simulink model "eight_point_dft"  (R2018a)
settings: Solver=VariableStepAuto  StartTime=0.0  StopTime=10.0  RelTol=1e-3
undefined symbols (not defined in the file): j
settings Model: Creator=eechris  LastModifiedBy=eechris

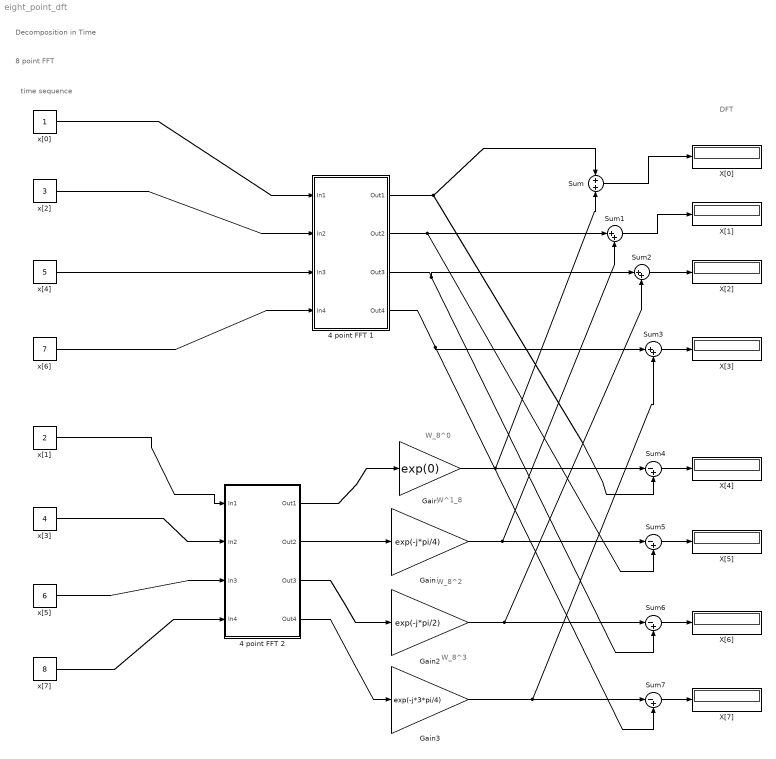
== system eight_point_dft ==
  note: Decomposition in Time
  note: W_8^3
  note: W_8^2
  note: W^1_8
  note: W_8^0
  note: time sequence
  note: DFT
  note: 8 point FFT
  4 point FFT 1 : Subsystem
  4 point FFT 2 : Subsystem
  Gain : Gain  Gain=exp(0)
  Gain1 : Gain  Gain=exp(-j*pi/4)
  Gain2 : Gain  Gain=exp(-j*pi/2)
  Gain3 : Gain  Gain=exp(-j*3*pi/4)
  Sum : Sum  Inputs=+|+
  Sum1 : Sum  Inputs=|++
  Sum2 : Sum  Inputs=|++
  Sum3 : Sum  Inputs=|++
  Sum{4..7} (4 alike) : Sum  Inputs=|-+
  X[0] : Display
  X[1] : Display
  X[2] : Display
  X[3] : Display
  X[4] : Display
  X[5] : Display
  X[6] : Display
  X[7] : Display
  x[0] : Constant
  x[1] : Constant  Value=2
  x[2] : Constant  Value=3
  x[3] : Constant  Value=4
  x[4] : Constant  Value=5
  x[5] : Constant  Value=6
  x[6] : Constant  Value=7
  x[7] : Constant  Value=8
  wires:
  x[0]/1 -> 4 point FFT 1/1(In1)
  x[7]/1 -> 4 point FFT 2/4(In4)
  Sum/1 -> X[0]/1
  4 point FFT 1/2(Out2) -> Sum5/2, Sum1/1
  Sum1/1 -> X[1]/1
  Sum3/1 -> X[3]/1
  Sum2/1 -> X[2]/1
  Sum4/1 -> X[4]/1
  Sum5/1 -> X[5]/1
  Sum6/1 -> X[6]/1
  Sum7/1 -> X[7]/1
  4 point FFT 2/1(Out1) -> Gain/1
  Gain/1 -> Sum/2, Sum4/1
  4 point FFT 2/2(Out2) -> Gain1/1
  Gain1/1 -> Sum1/2, Sum5/1
  Gain2/1 -> Sum2/2, Sum6/1
  4 point FFT 2/3(Out3) -> Gain2/1
  4 point FFT 2/4(Out4) -> Gain3/1
  Gain3/1 -> Sum3/2, Sum7/1
  4 point FFT 1/1(Out1) -> Sum4/2, Sum/1
  4 point FFT 1/3(Out3) -> Sum2/1, Sum6/2
  4 point FFT 1/4(Out4) -> Sum3/1, Sum7/2
  x[6]/1 -> 4 point FFT 1/4(In4)
  x[4]/1 -> 4 point FFT 1/3(In3)
  x[2]/1 -> 4 point FFT 1/2(In2)
  x[1]/1 -> 4 point FFT 2/1(In1)
  x[3]/1 -> 4 point FFT 2/2(In2)
  x[5]/1 -> 4 point FFT 2/3(In3)

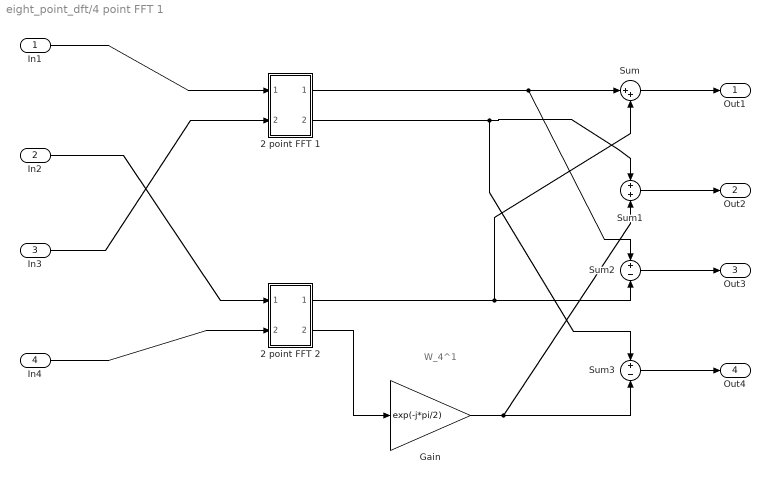
== system eight_point_dft/4 point FFT 1 ==
  note: W_4^1
  In1 : Inport
  In2 : Inport  Port=2
  In3 : Inport  Port=3
  In4 : Inport  Port=4
  2 point FFT 1 : Subsystem
  2 point FFT 2 : Subsystem
  Gain : Gain  Gain=exp(-j*pi/2)
  Sum : Sum  Inputs=|++
  Sum1 : Sum
  Sum2 : Sum  Inputs=+-
  Sum3 : Sum  Inputs=+-
  Out1 : Outport
  Out2 : Outport  Port=2
  Out3 : Outport  Port=3
  Out4 : Outport  Port=4
  wires:
  Sum3/1 -> Out4/1
  Gain/1 -> Sum1/2, Sum3/2
  In4/1 -> 2 point FFT 2/2(In2)
  In1/1 -> 2 point FFT 1/1(In1)
  2 point FFT 2/1(Out1) -> Sum2/2, Sum/2
  2 point FFT 2/2(Out2) -> Gain/1
  Sum1/1 -> Out2/1
  Sum/1 -> Out1/1
  Sum2/1 -> Out3/1
  2 point FFT 1/2(Out2) -> Sum1/1, Sum3/1
  2 point FFT 1/1(Out1) -> Sum2/1, Sum/1
  In2/1 -> 2 point FFT 2/1(In1)
  In3/1 -> 2 point FFT 1/2(In2)

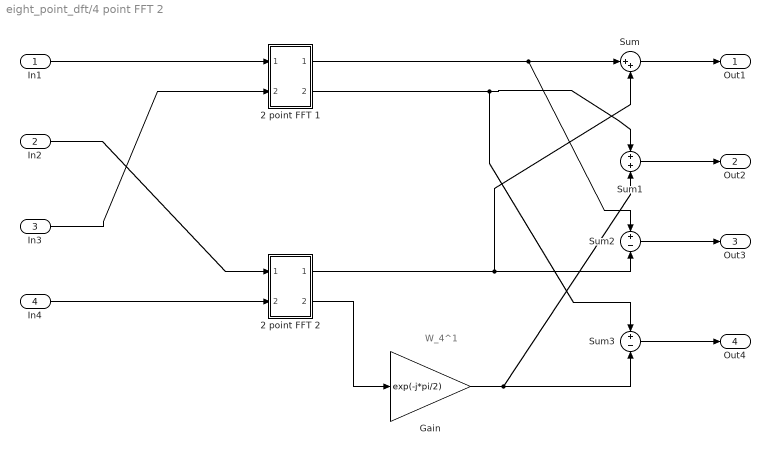
== system eight_point_dft/4 point FFT 2 ==
  note: W_4^1
  In1 : Inport
  In2 : Inport  Port=2
  In3 : Inport  Port=3
  In4 : Inport  Port=4
  2 point FFT 1 : Subsystem
  2 point FFT 2 : Subsystem
  Gain : Gain  Gain=exp(-j*pi/2)
  Sum : Sum  Inputs=|++
  Sum1 : Sum
  Sum2 : Sum  Inputs=+-
  Sum3 : Sum  Inputs=+-
  Out1 : Outport
  Out2 : Outport  Port=2
  Out3 : Outport  Port=3
  Out4 : Outport  Port=4
  wires:
  2 point FFT 1/1(Out1) -> Sum/1, Sum2/1
  2 point FFT 1/2(Out2) -> Sum3/1, Sum1/1
  Sum2/1 -> Out3/1
  Sum/1 -> Out1/1
  Sum1/1 -> Out2/1
  2 point FFT 2/2(Out2) -> Gain/1
  2 point FFT 2/1(Out1) -> Sum/2, Sum2/2
  In1/1 -> 2 point FFT 1/1(In1)
  In4/1 -> 2 point FFT 2/2(In2)
  Gain/1 -> Sum3/2, Sum1/2
  Sum3/1 -> Out4/1
  In3/1 -> 2 point FFT 1/2(In2)
  In2/1 -> 2 point FFT 2/1(In1)

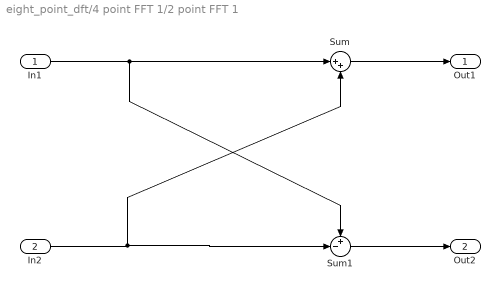
== system eight_point_dft/4 point FFT 1/2 point FFT 1 ==
  In1 : Inport
  In2 : Inport  Port=2
  Sum : Sum  Inputs=|++
  Sum1 : Sum  Inputs=+-|
  Out1 : Outport
  Out2 : Outport  Port=2
  wires:
  Sum/1 -> Out1/1
  In1/1 -> Sum1/1, Sum/1
  Sum1/1 -> Out2/1
  In2/1 -> Sum/2, Sum1/2

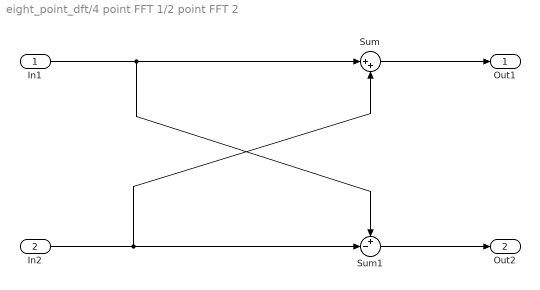
== system eight_point_dft/4 point FFT 1/2 point FFT 2 ==
  In1 : Inport
  In2 : Inport  Port=2
  Sum : Sum  Inputs=|++
  Sum1 : Sum  Inputs=+-|
  Out1 : Outport
  Out2 : Outport  Port=2
  wires:
  In2/1 -> Sum/2, Sum1/2
  Sum1/1 -> Out2/1
  In1/1 -> Sum/1, Sum1/1
  Sum/1 -> Out1/1

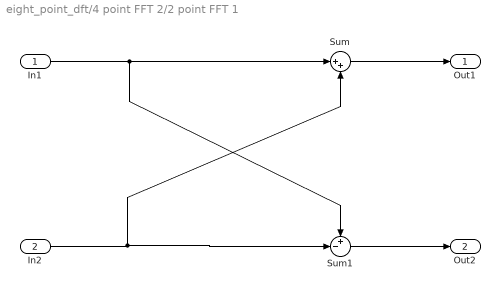
== system eight_point_dft/4 point FFT 2/2 point FFT 1 ==
  In1 : Inport
  In2 : Inport  Port=2
  Sum : Sum  Inputs=|++
  Sum1 : Sum  Inputs=+-|
  Out1 : Outport
  Out2 : Outport  Port=2
  wires:
  In2/1 -> Sum1/2, Sum/2
  Sum1/1 -> Out2/1
  In1/1 -> Sum/1, Sum1/1
  Sum/1 -> Out1/1

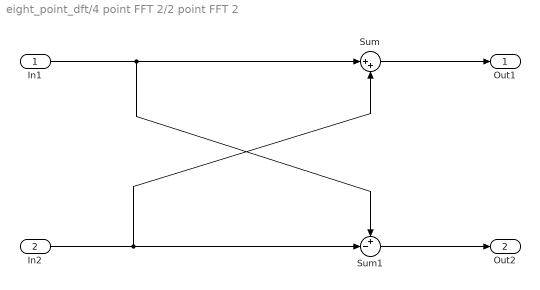
== system eight_point_dft/4 point FFT 2/2 point FFT 2 ==
  In1 : Inport
  In2 : Inport  Port=2
  Sum : Sum  Inputs=|++
  Sum1 : Sum  Inputs=+-|
  Out1 : Outport
  Out2 : Outport  Port=2
  wires:
  Sum/1 -> Out1/1
  In1/1 -> Sum1/1, Sum/1
  Sum1/1 -> Out2/1
  In2/1 -> Sum1/2, Sum/2
